simulink model "bh_4dof_LAGR_manipulator_CONTROL_PID"  (R2016b)
settings: Solver=ode15s  StartTime=0.0  StopTime=60  FixedStep=0.001  RelTol=1e-5  EnableMultiTasking=on
undefined symbols (not defined in the file or in its folder): b1_damp, b2_damp, b3_damp, b4_damp, g, Hz, L1x, L1y, L1z, L2x, L2y, L2z, L3x, L3y, L3z, mass1, mass2, mass3, mass4, Rturn, theta1_0, theta1_dot_0, theta2_0, theta2_dot_0, theta3_0, theta3_dot_0, theta4_0, theta4_dot_0, X, Y, Z
libraries: sm_lib x25, nesl_utility x17, simulink x9, simulink_extras x2
(part 2 of 3)

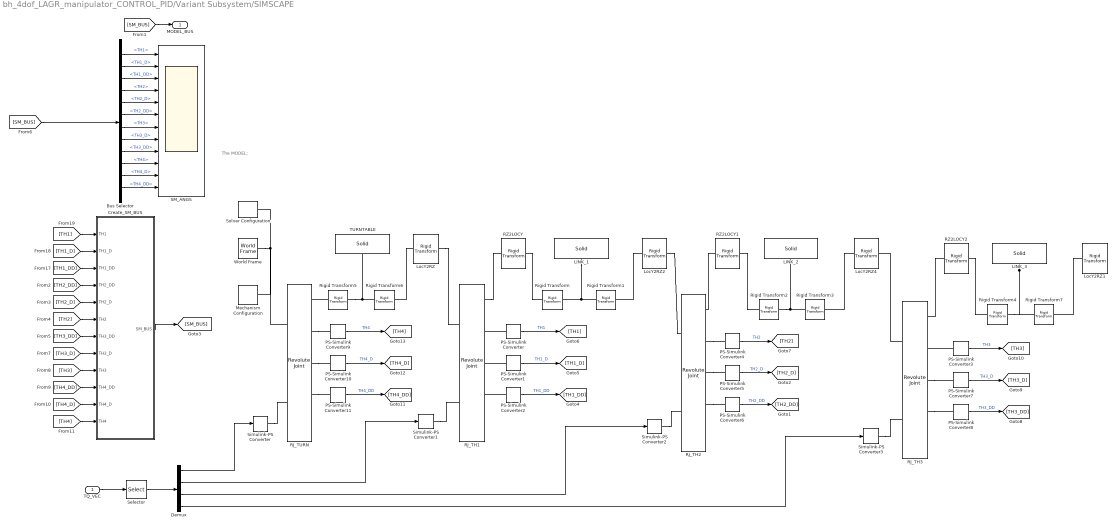
== system bh_4dof_LAGR_manipulator_CONTROL_PID/Variant Subsystem/SIMSCAPE ==
  note: The MODEL:
  TQ_VEC : Inport
  Bus Selector : BusSelector  OutputSignals=TH1,TH1_D,TH1_DD,TH2,TH2_D,TH2_DD,TH3,TH3_D,TH3_DD,TH4,TH4_D,TH4_DD
  Create_SM_BUS : Subsystem
  Demux : Demux
  LINK_1 : sm_lib/Body Elements/Solid  InertiaType=CalculateFromGeometry  Mass=1  MassUnits=kg  CenterOfMass=[0 0 0]  CenterOfMassUnits=m  MomentsOfInertia=[1 1 1]  MomentsOfInertiaUnits=kg*m^2  ProductsOfInertia=[0 0 0]  ProductsOfInertiaUnits=kg*m^2  DensityBased=on  Density=density  DensityUnits=kg/(m^3)  DoExposeReferenceFrame=on  SerializedFrames=<Frames/>  GraphicType=FromGeometry  MarkerShape=Sphere  MarkerSize=10  GraphicVisPropType=SimpleVisualProperties  GraphicDiffuseColor=[0.2 0.2 1.0]  GraphicSpecularColor=[0.5 0.5 0.5 1.0]  GraphicAmbientColor=[0.15 0.15 0.15 1.0]  GraphicEmissiveColor=[0.0 0.0 0.0 1.0]  GraphicShininess=75  GraphicOpacity=1.0  GeometryShape=Brick  RectangleSize=[1 1]  RectangleSizeUnits=m  BrickDimensions=[L1x, L1y, L1z ]  BrickDimensionUnits=m  CylinderRadius=1  CylinderRadiusUnits=m  CylinderLength=1  CylinderLengthUnits=m  SphereRadius=1  SphereRadiusUnits=m  EllipsoidRadii=[1 1 1]  EllipsoidRadiiUnits=m  ExtrusionCrossSection=[1 1; -1 1; -1 -1; 1 -1]  ExtrusionCrossSectionUnits=m  ExtrusionLength=1  ExtrusionLengthUnits=m  PolygonNumSides=3  PolygonOuterRadius=1  PolygonOuterRadiusUnits=m  ExtGeomFileType=STEP  ExtGeomFileUnits=m  RevolutionCrossSection=[1 1; 1 -1; 2 -1; 2 1]  RevolutionCrossSectionUnits=m  RevolutionExtent=Full  RevolutionAngle=180  RevolutionAngleUnits=deg
  LINK_2 : sm_lib/Body Elements/Solid  InertiaType=CalculateFromGeometry  Mass=1  MassUnits=kg  CenterOfMass=[0 0 0]  CenterOfMassUnits=m  MomentsOfInertia=[1 1 1]  MomentsOfInertiaUnits=kg*m^2  ProductsOfInertia=[0 0 0]  ProductsOfInertiaUnits=kg*m^2  DensityBased=on  Density=density  DensityUnits=kg/(m^3)  DoExposeReferenceFrame=on  SerializedFrames=<Frames/>  GraphicType=FromGeometry  MarkerShape=Sphere  MarkerSize=10  GraphicVisPropType=SimpleVisualProperties  GraphicDiffuseColor=[0.8 0.8 1.0]  GraphicSpecularColor=[0.5 0.5 0.5 1.0]  GraphicAmbientColor=[0.15 0.15 0.15 1.0]  GraphicEmissiveColor=[0.0 0.0 0.0 1.0]  GraphicShininess=75  GraphicOpacity=1.0  GeometryShape=Brick  RectangleSize=[1 1]  RectangleSizeUnits=m  BrickDimensions=[L2x, L2y, L2z ]  BrickDimensionUnits=m  CylinderRadius=1  CylinderRadiusUnits=m  CylinderLength=1  CylinderLengthUnits=m  SphereRadius=1  SphereRadiusUnits=m  EllipsoidRadii=[1 1 1]  EllipsoidRadiiUnits=m  ExtrusionCrossSection=[1 1; -1 1; -1 -1; 1 -1]  ExtrusionCrossSectionUnits=m  ExtrusionLength=1  ExtrusionLengthUnits=m  PolygonNumSides=3  PolygonOuterRadius=1  PolygonOuterRadiusUnits=m  ExtGeomFileType=STEP  ExtGeomFileUnits=m  RevolutionCrossSection=[1 1; 1 -1; 2 -1; 2 1]  RevolutionCrossSectionUnits=m  RevolutionExtent=Full  RevolutionAngle=180  RevolutionAngleUnits=deg
  LINK_3 : sm_lib/Body Elements/Solid  InertiaType=CalculateFromGeometry  Mass=1  MassUnits=kg  CenterOfMass=[0 0 0]  CenterOfMassUnits=m  MomentsOfInertia=[1 1 1]  MomentsOfInertiaUnits=kg*m^2  ProductsOfInertia=[0 0 0]  ProductsOfInertiaUnits=kg*m^2  DensityBased=on  Density=density  DensityUnits=kg/(m^3)  DoExposeReferenceFrame=on  SerializedFrames=<Frames/>  GraphicType=FromGeometry  MarkerShape=Sphere  MarkerSize=10  GraphicVisPropType=SimpleVisualProperties  GraphicDiffuseColor=[1.0 0.8 0.4]  GraphicSpecularColor=[0.5 0.5 0.5 1.0]  GraphicAmbientColor=[0.15 0.15 0.15 1.0]  GraphicEmissiveColor=[0.0 0.0 0.0 1.0]  GraphicShininess=75  GraphicOpacity=1.0  GeometryShape=Brick  RectangleSize=[1 1]  RectangleSizeUnits=m  BrickDimensions=[L3x, L3y, L3z ]  BrickDimensionUnits=m  CylinderRadius=1  CylinderRadiusUnits=m  CylinderLength=1  CylinderLengthUnits=m  SphereRadius=1  SphereRadiusUnits=m  EllipsoidRadii=[1 1 1]  EllipsoidRadiiUnits=m  ExtrusionCrossSection=[1 1; -1 1; -1 -1; 1 -1]  ExtrusionCrossSectionUnits=m  ExtrusionLength=1  ExtrusionLengthUnits=m  PolygonNumSides=3  PolygonOuterRadius=1  PolygonOuterRadiusUnits=m  ExtGeomFileType=STEP  ExtGeomFileUnits=m  RevolutionCrossSection=[1 1; 1 -1; 2 -1; 2 1]  RevolutionCrossSectionUnits=m  RevolutionExtent=Full  RevolutionAngle=180  RevolutionAngleUnits=deg
  LocY2RZ{,1..2,4} (4 alike) : sm_lib/Frames and Transforms/Rigid Transform  TranslationMethod=None  TranslationStandardOffset=Hz/2  TranslationLengthUnit=m  TranslationStandardAxis=+Z  TranslationCartesianOffset=[0 0 0]  TranslationROffset=0  TranslationROffsetUnits=m  TranslationZOffset=0  TranslationZOffsetUnits=m  TranslationThetaOffset=0  TranslationThetaOffsetUnits=deg  RotationMethod=AlignedAxes  RotationAngleUnits=deg  RotationStandardAxis=+Z  RotationAngle=0.0  RotationArbitraryAxis=[0 0 1]  FollAlignAxisA=+X  BaseAlignAxisA=+Y  FollAlignAxisB=+Y  BaseAlignAxisB=+Z  RotationSequenceAxes=FollowerAxes  RotationSequence=XYX  RotationSequenceAngles=[0 0 0]  RotationSequenceAnglesUnits=deg  RotationMatrix=[1 0 0; 0 1 0; 0 0 1]
  Mechanism Configuration : sm_lib/Utilities/Mechanism Configuration  UniformGravity=Constant  GravityVector=[0 0 -9.80665 ]  GravityUnits=m/s^2  LinearizationDelta=1e-4
  PS-Simulink Converter{,3..4,9} (4 alike) : nesl_utility/PS-Simulink Converter  PhysicalDomain=network_engine_domain  SubClassName=ps_output  LeftPortType=input  RightPortType=output  PseudoPeriodic=off  Frequencies=[]  Unit=rad  AffineConversion=off
  PS-Simulink Converter{1,5,7,10} (4 alike) : nesl_utility/PS-Simulink Converter  PhysicalDomain=network_engine_domain  SubClassName=ps_output  LeftPortType=input  RightPortType=output  PseudoPeriodic=off  Frequencies=[]  Unit=rad/s  AffineConversion=off
  PS-Simulink Converter{2,6,8,11} (4 alike) : nesl_utility/PS-Simulink Converter  PhysicalDomain=network_engine_domain  SubClassName=ps_output  LeftPortType=input  RightPortType=output  PseudoPeriodic=off  Frequencies=[]  Unit=rad/s^2  AffineConversion=off
  RJ_TH1 : sm_lib/Joints/Revolute Joint  SenseConstraintForce=on  SenseConstraintForceX=off  SenseConstraintForceY=off  SenseConstraintForceZ=off  SenseConstraintTorque=off  SenseConstraintTorqueX=off  SenseConstraintTorqueY=off  SenseConstraintTorqueZ=off  SenseTotalForce=off  SenseTotalForceX=off  SenseTotalForceY=off  SenseTotalForceZ=off  SenseTotalTorque=off  SenseTotalTorqueX=off  SenseTotalTorqueY=off  SenseTotalTorqueZ=off  CompositeWrenchDir=BaseOnFollower  CompositeWrenchFrame=BaseFrame  EquilibriumPosition=0  EquilibriumPositionUnits=deg  SpringStiffness=0  SpringStiffnessUnits=N*m/deg  DampingCoefficient=b1_damp  DampingCoefficientUnits=N*m/(rad/s)  TorqueActuationMode=InputTorque  MotionActuationMode=ComputedMotion  SensePosition=on  SenseVelocity=on  SenseAcceleration=on  SenseTorqueForce=off  PositionTargetSpecify=on  PositionTargetPriority=Low  PositionTargetValue=theta1_0  PositionTargetValueUnits=rad  VelocityTargetSpecify=on  VelocityTargetPriority=High  VelocityTargetValue=theta1_dot_0  VelocityTargetValueUnits=rad/s
      settings: AttributesFormatString=|
      | %<DampingCoefficient>
      | %<PositionTargetValue>
      | %<VelocityTargetValue>
  RJ_TH2 : sm_lib/Joints/Revolute Joint  SenseConstraintForce=on  SenseConstraintForceX=off  SenseConstraintForceY=off  SenseConstraintForceZ=off  SenseConstraintTorque=off  SenseConstraintTorqueX=off  SenseConstraintTorqueY=off  SenseConstraintTorqueZ=off  SenseTotalForce=off  SenseTotalForceX=off  SenseTotalForceY=off  SenseTotalForceZ=off  SenseTotalTorque=off  SenseTotalTorqueX=off  SenseTotalTorqueY=off  SenseTotalTorqueZ=off  CompositeWrenchDir=BaseOnFollower  CompositeWrenchFrame=BaseFrame  EquilibriumPosition=0  EquilibriumPositionUnits=deg  SpringStiffness=0  SpringStiffnessUnits=N*m/deg  DampingCoefficient=b2_damp  DampingCoefficientUnits=N*m/(rad/s)  TorqueActuationMode=InputTorque  MotionActuationMode=ComputedMotion  SensePosition=on  SenseVelocity=on  SenseAcceleration=on  SenseTorqueForce=off  PositionTargetSpecify=on  PositionTargetPriority=Low  PositionTargetValue=theta2_0  PositionTargetValueUnits=rad  VelocityTargetSpecify=on  VelocityTargetPriority=High  VelocityTargetValue=theta2_dot_0  VelocityTargetValueUnits=rad/s
      settings: AttributesFormatString=|
      | %<DampingCoefficient>
      | %<PositionTargetValue>
      | %<VelocityTargetValue>
  RJ_TH3 : sm_lib/Joints/Revolute Joint  SenseConstraintForce=on  SenseConstraintForceX=off  SenseConstraintForceY=off  SenseConstraintForceZ=off  SenseConstraintTorque=off  SenseConstraintTorqueX=off  SenseConstraintTorqueY=off  SenseConstraintTorqueZ=off  SenseTotalForce=off  SenseTotalForceX=off  SenseTotalForceY=off  SenseTotalForceZ=off  SenseTotalTorque=off  SenseTotalTorqueX=off  SenseTotalTorqueY=off  SenseTotalTorqueZ=off  CompositeWrenchDir=BaseOnFollower  CompositeWrenchFrame=BaseFrame  EquilibriumPosition=0  EquilibriumPositionUnits=deg  SpringStiffness=0  SpringStiffnessUnits=N*m/deg  DampingCoefficient=b3_damp  DampingCoefficientUnits=N*m/(rad/s)  TorqueActuationMode=InputTorque  MotionActuationMode=ComputedMotion  SensePosition=on  SenseVelocity=on  SenseAcceleration=on  SenseTorqueForce=off  PositionTargetSpecify=on  PositionTargetPriority=Low  PositionTargetValue=theta3_0  PositionTargetValueUnits=rad  VelocityTargetSpecify=on  VelocityTargetPriority=High  VelocityTargetValue=theta3_dot_0  VelocityTargetValueUnits=rad/s
      settings: AttributesFormatString=|
      | %<DampingCoefficient>
      | %<PositionTargetValue>
      | %<VelocityTargetValue>
  RJ_TURN : sm_lib/Joints/Revolute Joint  SenseConstraintForce=on  SenseConstraintForceX=off  SenseConstraintForceY=off  SenseConstraintForceZ=off  SenseConstraintTorque=off  SenseConstraintTorqueX=off  SenseConstraintTorqueY=off  SenseConstraintTorqueZ=off  SenseTotalForce=off  SenseTotalForceX=off  SenseTotalForceY=off  SenseTotalForceZ=off  SenseTotalTorque=off  SenseTotalTorqueX=off  SenseTotalTorqueY=off  SenseTotalTorqueZ=off  CompositeWrenchDir=BaseOnFollower  CompositeWrenchFrame=BaseFrame  EquilibriumPosition=0  EquilibriumPositionUnits=deg  SpringStiffness=0  SpringStiffnessUnits=N*m/deg  DampingCoefficient=b4_damp  DampingCoefficientUnits=N*m/(rad/s)  TorqueActuationMode=InputTorque  MotionActuationMode=ComputedMotion  SensePosition=on  SenseVelocity=on  SenseAcceleration=on  SenseTorqueForce=off  PositionTargetSpecify=on  PositionTargetPriority=Low  PositionTargetValue=theta4_0  PositionTargetValueUnits=rad  VelocityTargetSpecify=on  VelocityTargetPriority=High  VelocityTargetValue=theta4_dot_0  VelocityTargetValueUnits=rad/s
      settings: AttributesFormatString=|
      | %<DampingCoefficient>
      | %<PositionTargetValue>
      | %<VelocityTargetValue>
  RZ2LOCY : sm_lib/Frames and Transforms/Rigid Transform  TranslationMethod=None  TranslationStandardOffset=Hz/2  TranslationLengthUnit=m  TranslationStandardAxis=+Z  TranslationCartesianOffset=[0 0 0]  TranslationROffset=0  TranslationROffsetUnits=m  TranslationZOffset=0  TranslationZOffsetUnits=m  TranslationThetaOffset=0  TranslationThetaOffsetUnits=deg  RotationMethod=AlignedAxes  RotationAngleUnits=deg  RotationStandardAxis=+Z  RotationAngle=0.0  RotationArbitraryAxis=[0 0 1]  FollAlignAxisA=+Y  BaseAlignAxisA=+X  FollAlignAxisB=+X  BaseAlignAxisB=+Z  RotationSequenceAxes=FollowerAxes  RotationSequence=XYX  RotationSequenceAngles=[0 0 0]  RotationSequenceAnglesUnits=deg  RotationMatrix=[1 0 0; 0 1 0; 0 0 1]
  RZ2LOCY1 : sm_lib/Frames and Transforms/Rigid Transform  TranslationMethod=None  TranslationStandardOffset=Hz/2  TranslationLengthUnit=m  TranslationStandardAxis=+Z  TranslationCartesianOffset=[0 0 0]  TranslationROffset=0  TranslationROffsetUnits=m  TranslationZOffset=0  TranslationZOffsetUnits=m  TranslationThetaOffset=0  TranslationThetaOffsetUnits=deg  RotationMethod=AlignedAxes  RotationAngleUnits=deg  RotationStandardAxis=+Z  RotationAngle=0.0  RotationArbitraryAxis=[0 0 1]  FollAlignAxisA=+Y  BaseAlignAxisA=+X  FollAlignAxisB=+X  BaseAlignAxisB=+Z  RotationSequenceAxes=FollowerAxes  RotationSequence=XYX  RotationSequenceAngles=[0 0 0]  RotationSequenceAnglesUnits=deg  RotationMatrix=[1 0 0; 0 1 0; 0 0 1]
  RZ2LOCY2 : sm_lib/Frames and Transforms/Rigid Transform  TranslationMethod=None  TranslationStandardOffset=Hz/2  TranslationLengthUnit=m  TranslationStandardAxis=+Z  TranslationCartesianOffset=[0 0 0]  TranslationROffset=0  TranslationROffsetUnits=m  TranslationZOffset=0  TranslationZOffsetUnits=m  TranslationThetaOffset=0  TranslationThetaOffsetUnits=deg  RotationMethod=AlignedAxes  RotationAngleUnits=deg  RotationStandardAxis=+Z  RotationAngle=0.0  RotationArbitraryAxis=[0 0 1]  FollAlignAxisA=+Y  BaseAlignAxisA=+X  FollAlignAxisB=+X  BaseAlignAxisB=+Z  RotationSequenceAxes=FollowerAxes  RotationSequence=XYX  RotationSequenceAngles=[0 0 0]  RotationSequenceAnglesUnits=deg  RotationMatrix=[1 0 0; 0 1 0; 0 0 1]
  Rigid Transform : sm_lib/Frames and Transforms/Rigid Transform  TranslationMethod=StandardAxis  TranslationStandardOffset=L1y/2  TranslationLengthUnit=m  TranslationStandardAxis=+Y  TranslationCartesianOffset=[0 0 0]  TranslationROffset=0  TranslationROffsetUnits=m  TranslationZOffset=0  TranslationZOffsetUnits=m  TranslationThetaOffset=0  TranslationThetaOffsetUnits=deg  RotationMethod=None  RotationAngleUnits=deg  RotationStandardAxis=+Z  RotationAngle=0.0  RotationArbitraryAxis=[0 0 1]  FollAlignAxisA=+X  BaseAlignAxisA=+Y  FollAlignAxisB=+Y  BaseAlignAxisB=+Z  RotationSequenceAxes=FollowerAxes  RotationSequence=XYX  RotationSequenceAngles=[0 0 0]  RotationSequenceAnglesUnits=deg  RotationMatrix=[1 0 0; 0 1 0; 0 0 1]
  Rigid Transform1 : sm_lib/Frames and Transforms/Rigid Transform  TranslationMethod=StandardAxis  TranslationStandardOffset=L1y/2  TranslationLengthUnit=m  TranslationStandardAxis=+Y  TranslationCartesianOffset=[0 0 0]  TranslationROffset=0  TranslationROffsetUnits=m  TranslationZOffset=0  TranslationZOffsetUnits=m  TranslationThetaOffset=0  TranslationThetaOffsetUnits=deg  RotationMethod=None  RotationAngleUnits=deg  RotationStandardAxis=+Z  RotationAngle=0.0  RotationArbitraryAxis=[0 0 1]  FollAlignAxisA=+X  BaseAlignAxisA=+Y  FollAlignAxisB=+Y  BaseAlignAxisB=+Z  RotationSequenceAxes=FollowerAxes  RotationSequence=XYX  RotationSequenceAngles=[0 0 0]  RotationSequenceAnglesUnits=deg  RotationMatrix=[1 0 0; 0 1 0; 0 0 1]
  Rigid Transform2 : sm_lib/Frames and Transforms/Rigid Transform  TranslationMethod=StandardAxis  TranslationStandardOffset=L2y/2  TranslationLengthUnit=m  TranslationStandardAxis=+Y  TranslationCartesianOffset=[0 0 0]  TranslationROffset=0  TranslationROffsetUnits=m  TranslationZOffset=0  TranslationZOffsetUnits=m  TranslationThetaOffset=0  TranslationThetaOffsetUnits=deg  RotationMethod=None  RotationAngleUnits=deg  RotationStandardAxis=+Z  RotationAngle=0.0  RotationArbitraryAxis=[0 0 1]  FollAlignAxisA=+X  BaseAlignAxisA=+Y  FollAlignAxisB=+Y  BaseAlignAxisB=+Z  RotationSequenceAxes=FollowerAxes  RotationSequence=XYX  RotationSequenceAngles=[0 0 0]  RotationSequenceAnglesUnits=deg  RotationMatrix=[1 0 0; 0 1 0; 0 0 1]
  Rigid Transform3 : sm_lib/Frames and Transforms/Rigid Transform  TranslationMethod=StandardAxis  TranslationStandardOffset=L2y/2  TranslationLengthUnit=m  TranslationStandardAxis=+Y  TranslationCartesianOffset=[0 0 0]  TranslationROffset=0  TranslationROffsetUnits=m  TranslationZOffset=0  TranslationZOffsetUnits=m  TranslationThetaOffset=0  TranslationThetaOffsetUnits=deg  RotationMethod=None  RotationAngleUnits=deg  RotationStandardAxis=+Z  RotationAngle=0.0  RotationArbitraryAxis=[0 0 1]  FollAlignAxisA=+X  BaseAlignAxisA=+Y  FollAlignAxisB=+Y  BaseAlignAxisB=+Z  RotationSequenceAxes=FollowerAxes  RotationSequence=XYX  RotationSequenceAngles=[0 0 0]  RotationSequenceAnglesUnits=deg  RotationMatrix=[1 0 0; 0 1 0; 0 0 1]
  Rigid Transform4 : sm_lib/Frames and Transforms/Rigid Transform  TranslationMethod=StandardAxis  TranslationStandardOffset=L3y/2  TranslationLengthUnit=m  TranslationStandardAxis=+Y  TranslationCartesianOffset=[0 0 0]  TranslationROffset=0  TranslationROffsetUnits=m  TranslationZOffset=0  TranslationZOffsetUnits=m  TranslationThetaOffset=0  TranslationThetaOffsetUnits=deg  RotationMethod=None  RotationAngleUnits=deg  RotationStandardAxis=+Z  RotationAngle=0.0  RotationArbitraryAxis=[0 0 1]  FollAlignAxisA=+X  BaseAlignAxisA=+Y  FollAlignAxisB=+Y  BaseAlignAxisB=+Z  RotationSequenceAxes=FollowerAxes  RotationSequence=XYX  RotationSequenceAngles=[0 0 0]  RotationSequenceAnglesUnits=deg  RotationMatrix=[1 0 0; 0 1 0; 0 0 1]
  Rigid Transform5 : sm_lib/Frames and Transforms/Rigid Transform  TranslationMethod=StandardAxis  TranslationStandardOffset=Hz/2  TranslationLengthUnit=m  TranslationStandardAxis=-Z  TranslationCartesianOffset=[0 0 0]  TranslationROffset=0  TranslationROffsetUnits=m  TranslationZOffset=0  TranslationZOffsetUnits=m  TranslationThetaOffset=0  TranslationThetaOffsetUnits=deg  RotationMethod=None  RotationAngleUnits=deg  RotationStandardAxis=+Z  RotationAngle=0.0  RotationArbitraryAxis=[0 0 1]  FollAlignAxisA=+X  BaseAlignAxisA=+Y  FollAlignAxisB=+Y  BaseAlignAxisB=+Z  RotationSequenceAxes=FollowerAxes  RotationSequence=XYX  RotationSequenceAngles=[0 0 0]  RotationSequenceAnglesUnits=deg  RotationMatrix=[1 0 0; 0 1 0; 0 0 1]
  Rigid Transform6 : sm_lib/Frames and Transforms/Rigid Transform  TranslationMethod=StandardAxis  TranslationStandardOffset=Hz/2  TranslationLengthUnit=m  TranslationStandardAxis=+Z  TranslationCartesianOffset=[0 0 0]  TranslationROffset=0  TranslationROffsetUnits=m  TranslationZOffset=0  TranslationZOffsetUnits=m  TranslationThetaOffset=0  TranslationThetaOffsetUnits=deg  RotationMethod=None  RotationAngleUnits=deg  RotationStandardAxis=+Z  RotationAngle=0.0  RotationArbitraryAxis=[0 0 1]  FollAlignAxisA=+X  BaseAlignAxisA=+Y  FollAlignAxisB=+Y  BaseAlignAxisB=+Z  RotationSequenceAxes=FollowerAxes  RotationSequence=XYX  RotationSequenceAngles=[0 0 0]  RotationSequenceAnglesUnits=deg  RotationMatrix=[1 0 0; 0 1 0; 0 0 1]
  Rigid Transform7 : sm_lib/Frames and Transforms/Rigid Transform  TranslationMethod=StandardAxis  TranslationStandardOffset=L3y/2  TranslationLengthUnit=m  TranslationStandardAxis=+Y  TranslationCartesianOffset=[0 0 0]  TranslationROffset=0  TranslationROffsetUnits=m  TranslationZOffset=0  TranslationZOffsetUnits=m  TranslationThetaOffset=0  TranslationThetaOffsetUnits=deg  RotationMethod=None  RotationAngleUnits=deg  RotationStandardAxis=+Z  RotationAngle=0.0  RotationArbitraryAxis=[0 0 1]  FollAlignAxisA=+X  BaseAlignAxisA=+Y  FollAlignAxisB=+Y  BaseAlignAxisB=+Z  RotationSequenceAxes=FollowerAxes  RotationSequence=XYX  RotationSequenceAngles=[0 0 0]  RotationSequenceAnglesUnits=deg  RotationMatrix=[1 0 0; 0 1 0; 0 0 1]
  SM_ANGS : Scope  NumInputPorts=12
  Selector : Selector  InputPortWidth=4  IndexOptions=Index vector (dialog)  Indices=[4 1 2 3]  OutputSizes=1
  Simulink-PS Converter{,1..3} (4 alike) : nesl_utility/Simulink-PS Converter  PhysicalDomain=network_engine_domain  SubClassName=ps_input  LeftPortType=input  RightPortType=output  PseudoPeriodic=off  Frequencies=[]  NoiseDistribution=none  NoiseParameters=[]  Unit=N*m  AffineConversion=off  InputFiltering=off  SimscapeFilterOrder=1  InputFilterTimeConstant=0.001  UdotUserProvided=1
  Solver Configuration : nesl_utility/Solver Configuration  PhysicalDomain=network_engine_domain  SubClassName=solver  LeftPortType=input  RightPortType=generic  Accelerate=off  Tones=[]  Harmonics=[]  SimulateNoise=off  Profile=off  UseLocalSampling=off  EnableSwitchedLinearOptims=on  FrequencyDomain=off  UseCCode=off  RelTol=0.001  AbsTol=1e-06  MinStep=1e-09  ToWorkspace=off  RevertToSquareIcSolve=off  NumHomotopyIterations=100  PhasorMode=off  PhasorModeNumHarmonics=1  OverrideAbsTol=off  DoDC=off  ResidualTolerance=1e-09  UseLocalSolver=off  LocalSolverChoice=NE_TRAPEZOIDAL_ADVANCER  LocalSolverSampleTime=0.01  DoFixedCost=off  MaxNonlinIter=3  MaxModeIter=2  LinearAlgebra=Sparse  DelaysMemoryBudget=1024  AutomaticFiltering=off  FilteringTimeConstant=0.001
  TURNTABLE : sm_lib/Body Elements/Solid  InertiaType=CalculateFromGeometry  Mass=1  MassUnits=kg  CenterOfMass=[0 0 0]  CenterOfMassUnits=m  MomentsOfInertia=[1 1 1]  MomentsOfInertiaUnits=kg*m^2  ProductsOfInertia=[0 0 0]  ProductsOfInertiaUnits=kg*m^2  DensityBased=on  Density=1000  DensityUnits=kg/(m^3)  DoExposeReferenceFrame=on  SerializedFrames=<Frames/>  GraphicType=FromGeometry  MarkerShape=Sphere  MarkerSize=10  GraphicVisPropType=SimpleVisualProperties  GraphicDiffuseColor=[1.0 1.0 0.2]  GraphicSpecularColor=[0.5 0.5 0.5 1.0]  GraphicAmbientColor=[0.15 0.15 0.15 1.0]  GraphicEmissiveColor=[0.0 0.0 0.0 1.0]  GraphicShininess=75  GraphicOpacity=1.0  GeometryShape=Cylinder  RectangleSize=[1 1]  RectangleSizeUnits=m  BrickDimensions=[1 1 1]  BrickDimensionUnits=m  CylinderRadius=Rturn  CylinderRadiusUnits=m  CylinderLength=Hz  CylinderLengthUnits=m  SphereRadius=1  SphereRadiusUnits=m  EllipsoidRadii=[1 1 1]  EllipsoidRadiiUnits=m  ExtrusionCrossSection=[1 1; -1 1; -1 -1; 1 -1]  ExtrusionCrossSectionUnits=m  ExtrusionLength=1  ExtrusionLengthUnits=m  PolygonNumSides=3  PolygonOuterRadius=1  PolygonOuterRadiusUnits=m  ExtGeomFileType=STEP  ExtGeomFileUnits=m  RevolutionCrossSection=[1 1; 1 -1; 2 -1; 2 1]  RevolutionCrossSectionUnits=m  RevolutionExtent=Full  RevolutionAngle=180  RevolutionAngleUnits=deg
  World Frame : sm_lib/Frames and Transforms/World Frame
  MODEL_BUS : Outport
  wires:
  [SM_BUS] -> MODEL_BUS/1
  [TH2_D] -> Create_SM_BUS/5(TH2_D)
  [TH1_D] -> Create_SM_BUS/2(TH1_D)
  [TH2_DD] -> Create_SM_BUS/4(TH2_DD)
  [TH2] -> Create_SM_BUS/6(TH2)
  [TH1_DD] -> Create_SM_BUS/3(TH1_DD)
  [TH1] -> Create_SM_BUS/1(TH1)
  Create_SM_BUS/1(SM_BUS) -> [SM_BUS]
  Bus Selector/2 -> SM_ANGS/2  "<TH1_D>"
  Bus Selector/3 -> SM_ANGS/3  "<TH1_DD>"
  Bus Selector/1 -> SM_ANGS/1  "<TH1>"
  Bus Selector/4 -> SM_ANGS/4  "<TH2>"
  Bus Selector/5 -> SM_ANGS/5  "<TH2_D>"
  Bus Selector/6 -> SM_ANGS/6  "<TH2_DD>"
  Bus Selector/7 -> SM_ANGS/7  "<TH3>"
  Bus Selector/8 -> SM_ANGS/8  "<TH3_D>"
  Bus Selector/9 -> SM_ANGS/9  "<TH3_DD>"
  [TH3_DD] -> Create_SM_BUS/7(TH3_DD)
  [TH3_D] -> Create_SM_BUS/8(TH3_D)
  [TH3] -> Create_SM_BUS/9(TH3)
  PS-Simulink Converter/1 -> [TH1]  "TH1"
  PS-Simulink Converter2/1 -> [TH1_DD]  "TH1_DD"
  PS-Simulink Converter1/1 -> [TH1_D]  "TH1_D"
  PS-Simulink Converter4/1 -> [TH2]  "TH2"
  PS-Simulink Converter6/1 -> [TH2_DD]  "TH2_DD"
  PS-Simulink Converter5/1 -> [TH2_D]  "TH2_D"
  PS-Simulink Converter3/1 -> [TH3]  "TH3"
  PS-Simulink Converter8/1 -> [TH3_DD]  "TH3_DD"
  PS-Simulink Converter7/1 -> [TH3_D]  "TH3_D"
  PS-Simulink Converter9/1 -> [TH4]  "TH4"
  PS-Simulink Converter11/1 -> [TH4_DD]  "TH4_DD"
  PS-Simulink Converter10/1 -> [TH4_D]  "TH4_D"
  [TH4_DD] -> Create_SM_BUS/10(TH4_DD)
  [TH4_D] -> Create_SM_BUS/11(TH4_D)
  [TH4] -> Create_SM_BUS/12(TH4)
  Bus Selector/12 -> SM_ANGS/12  "<TH4_DD>"
  Bus Selector/11 -> SM_ANGS/11  "<TH4_D>"
  Bus Selector/10 -> SM_ANGS/10  "<TH4>"
  [SM_BUS] -> Bus Selector/1
  Demux/1 -> Simulink-PS Converter/1
  Demux/2 -> Simulink-PS Converter1/1
  Demux/3 -> Simulink-PS Converter2/1
  Demux/4 -> Simulink-PS Converter3/1
  TQ_VEC/1 -> Selector/1
  Selector/1 -> Demux/1
  connections:
  World Frame/RConn1 -- RJ_TURN/LConn1 -- Mechanism Configuration/RConn1 -- Solver Configuration/RConn1
  PS-Simulink Converter1/LConn1 -- RJ_TH1/RConn3
  PS-Simulink Converter2/LConn1 -- RJ_TH1/RConn4
  PS-Simulink Converter/LConn1 -- RJ_TH1/RConn2
  Rigid Transform5/LConn1 -- RJ_TURN/RConn1
  Rigid Transform5/RConn1 -- Rigid Transform6/LConn1 -- TURNTABLE/RConn1
  LocY2RZ/LConn1 -- Rigid Transform6/RConn1
  LocY2RZ/RConn1 -- RJ_TH1/LConn1
  Rigid Transform1/LConn1 -- LINK_1/RConn1 -- Rigid Transform/RConn1
  LocY2RZ2/LConn1 -- Rigid Transform1/RConn1
  LocY2RZ2/RConn1 -- RJ_TH2/LConn1
  RZ2LOCY1/LConn1 -- RJ_TH2/RConn1
  Rigid Transform2/RConn1 -- Rigid Transform3/LConn1 -- LINK_2/RConn1
  LocY2RZ4/LConn1 -- Rigid Transform3/RConn1
  RJ_TH1/RConn1 -- RZ2LOCY/LConn1
  RZ2LOCY/RConn1 -- Rigid Transform/LConn1
  RZ2LOCY1/RConn1 -- Rigid Transform2/LConn1
  RJ_TH3/LConn1 -- LocY2RZ4/RConn1
  LINK_3/RConn1 -- Rigid Transform7/LConn1 -- Rigid Transform4/RConn1
  LocY2RZ1/LConn1 -- Rigid Transform7/RConn1
  RZ2LOCY2/RConn1 -- Rigid Transform4/LConn1
  RZ2LOCY2/LConn1 -- RJ_TH3/RConn1
  RJ_TH2/RConn3 -- PS-Simulink Converter5/LConn1
  RJ_TH2/RConn2 -- PS-Simulink Converter4/LConn1
  RJ_TH2/RConn4 -- PS-Simulink Converter6/LConn1
  PS-Simulink Converter3/LConn1 -- RJ_TH3/RConn2
  RJ_TH3/RConn3 -- PS-Simulink Converter7/LConn1
  RJ_TH3/RConn4 -- PS-Simulink Converter8/LConn1
  RJ_TURN/RConn4 -- PS-Simulink Converter11/LConn1
  RJ_TURN/RConn3 -- PS-Simulink Converter10/LConn1
  RJ_TURN/RConn2 -- PS-Simulink Converter9/LConn1
  Simulink-PS Converter/RConn1 -- RJ_TURN/LConn2
  Simulink-PS Converter2/RConn1 -- RJ_TH2/LConn2
  Simulink-PS Converter3/RConn1 -- RJ_TH3/LConn2
  Simulink-PS Converter1/RConn1 -- RJ_TH1/LConn2

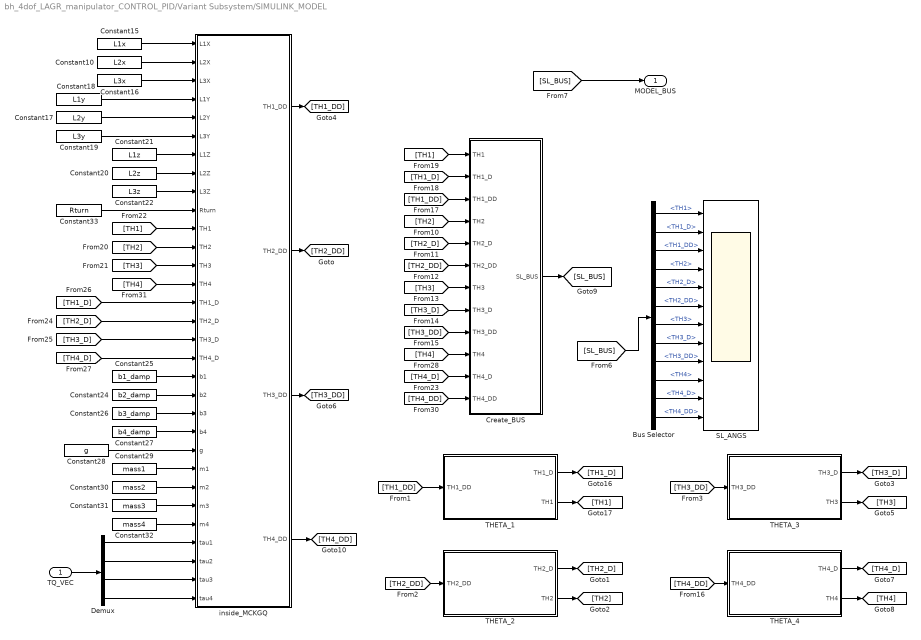
== system bh_4dof_LAGR_manipulator_CONTROL_PID/Variant Subsystem/SIMULINK_MODEL ==
  TQ_VEC : Inport
  Bus Selector : BusSelector  OutputSignals=TH1,TH1_D,TH1_DD,TH2,TH2_D,TH2_DD,TH3,TH3_D,TH3_DD,TH4,TH4_D,TH4_DD
  Constant10 : Constant  Value=L2x
  Constant15 : Constant  Value=L1x
  Constant16 : Constant  Value=L3x
  Constant17 : Constant  Value=L2y
  Constant18 : Constant  Value=L1y
  Constant19 : Constant  Value=L3y
  Constant20 : Constant  Value=L2z
  Constant21 : Constant  Value=L1z
  Constant22 : Constant  Value=L3z
  Constant24 : Constant  Value=b2_damp
  Constant25 : Constant  Value=b1_damp
  Constant26 : Constant  Value=b3_damp
  Constant27 : Constant  Value=b4_damp
  Constant28 : Constant  Value=g
  Constant29 : Constant  Value=mass1
  Constant30 : Constant  Value=mass2
  Constant31 : Constant  Value=mass3
  Constant32 : Constant  Value=mass4
  Constant33 : Constant  Value=Rturn
  Create_BUS : Subsystem
  Demux : Demux
  SL_ANGS : Scope  NumInputPorts=12
  THETA_1 : Subsystem
  THETA_2 : Subsystem
  THETA_3 : Subsystem
  THETA_4 : Subsystem
  inside_MCKGQ : Subsystem
  MODEL_BUS : Outport
  wires:
  [SL_BUS] -> Bus Selector/1
  Create_BUS/1(SL_BUS) -> [SL_BUS]
  Bus Selector/2 -> SL_ANGS/2  "<TH1_D>"
  Bus Selector/3 -> SL_ANGS/3  "<TH1_DD>"
  Bus Selector/1 -> SL_ANGS/1  "<TH1>"
  Bus Selector/4 -> SL_ANGS/4  "<TH2>"
  Bus Selector/5 -> SL_ANGS/5  "<TH2_D>"
  Bus Selector/6 -> SL_ANGS/6  "<TH2_DD>"
  Bus Selector/7 -> SL_ANGS/7  "<TH3>"
  Bus Selector/8 -> SL_ANGS/8  "<TH3_D>"
  Bus Selector/9 -> SL_ANGS/9  "<TH3_DD>"
  [TH2_DD] -> THETA_2/1(TH2_DD)
  THETA_2/2(TH2) -> [TH2]
  THETA_2/1(TH2_D) -> [TH2_D]
  [TH1_DD] -> THETA_1/1(TH1_DD)
  THETA_1/1(TH1_D) -> [TH1_D]
  THETA_1/2(TH1) -> [TH1]
  inside_MCKGQ/2(TH2_DD) -> [TH2_DD]
  [TH3_DD] -> THETA_3/1(TH3_DD)
  THETA_3/2(TH3) -> [TH3]
  THETA_3/1(TH3_D) -> [TH3_D]
  inside_MCKGQ/1(TH1_DD) -> [TH1_DD]
  inside_MCKGQ/3(TH3_DD) -> [TH3_DD]
  [TH3_DD] -> Create_BUS/9(TH3_DD)
  [TH1] -> Create_BUS/1(TH1)
  [TH1_D] -> Create_BUS/2(TH1_D)
  [TH1_DD] -> Create_BUS/3(TH1_DD)
  [TH2] -> Create_BUS/4(TH2)
  [TH2_D] -> Create_BUS/5(TH2_D)
  [TH2_DD] -> Create_BUS/6(TH2_DD)
  [TH3] -> Create_BUS/7(TH3)
  [TH3_D] -> Create_BUS/8(TH3_D)
  [TH4_DD] -> THETA_4/1(TH4_DD)
  THETA_4/2(TH4) -> [TH4]
  THETA_4/1(TH4_D) -> [TH4_D]
  [TH2] -> inside_MCKGQ/12(TH2)
  [TH3] -> inside_MCKGQ/13(TH3)
  [TH1] -> inside_MCKGQ/11(TH1)
  Constant10/1 -> inside_MCKGQ/2(L2X)
  Constant16/1 -> inside_MCKGQ/3(L3X)
  Constant15/1 -> inside_MCKGQ/1(L1X)
  Constant19/1 -> inside_MCKGQ/6(L3Y)
  Constant17/1 -> inside_MCKGQ/5(L2Y)
  Constant18/1 -> inside_MCKGQ/4(L1Y)
  Constant22/1 -> inside_MCKGQ/9(L3Z)
  Constant20/1 -> inside_MCKGQ/8(L2Z)
  Constant21/1 -> inside_MCKGQ/7(L1Z)
  [TH1_D] -> inside_MCKGQ/15(TH1_D)
  [TH2_D] -> inside_MCKGQ/16(TH2_D)
  [TH3_D] -> inside_MCKGQ/17(TH3_D)
  [TH4_D] -> inside_MCKGQ/18(TH4_D)
  Constant25/1 -> inside_MCKGQ/19(b1)
  Constant24/1 -> inside_MCKGQ/20(b2)
  Constant26/1 -> inside_MCKGQ/21(b3)
  Constant27/1 -> inside_MCKGQ/22(b4)
  Constant28/1 -> inside_MCKGQ/23(g)
  Constant29/1 -> inside_MCKGQ/24(m1)
  Constant30/1 -> inside_MCKGQ/25(m2)
  Constant31/1 -> inside_MCKGQ/26(m3)
  Constant32/1 -> inside_MCKGQ/27(m4)
  Constant33/1 -> inside_MCKGQ/10(Rturn)
  [TH4_D] -> Create_BUS/11(TH4_D)
  [TH4_DD] -> Create_BUS/12(TH4_DD)
  [TH4] -> Create_BUS/10(TH4)
  [TH4] -> inside_MCKGQ/14(TH4)
  inside_MCKGQ/4(TH4_DD) -> [TH4_DD]
  Bus Selector/10 -> SL_ANGS/10  "<TH4>"
  Bus Selector/11 -> SL_ANGS/11  "<TH4_D>"
  Bus Selector/12 -> SL_ANGS/12  "<TH4_DD>"
  [SL_BUS] -> MODEL_BUS/1
  Demux/1 -> inside_MCKGQ/28(tau1)
  Demux/2 -> inside_MCKGQ/29(tau2)
  Demux/3 -> inside_MCKGQ/30(tau3)
  Demux/4 -> inside_MCKGQ/31(tau4)
  TQ_VEC/1 -> Demux/1

== system bh_4dof_LAGR_manipulator_CONTROL_PID/Create_PLANT_BUS/Subsystem1/Subsystem1 ==
  mg_signed : Inport
  Constant : Constant  Value=0
  Mux : Mux  Inputs=3
  Reshape : Reshape  OutputDimensionality=Column vector (2-D)
  COL : Outport
  wires:
  mg_signed/1 -> Mux/3
  Constant/1 -> Mux/2, Mux/1
  Mux/1 -> Reshape/1
  Reshape/1 -> COL/1

== system bh_4dof_LAGR_manipulator_CONTROL_PID/Create_PLANT_BUS/Subsystem1/Subsystem2 ==
  mg_signed : Inport
  Constant : Constant  Value=0
  Mux : Mux  Inputs=3
  Reshape : Reshape  OutputDimensionality=Column vector (2-D)
  COL : Outport
  wires:
  mg_signed/1 -> Mux/3
  Constant/1 -> Mux/2, Mux/1
  Mux/1 -> Reshape/1
  Reshape/1 -> COL/1

== system bh_4dof_LAGR_manipulator_CONTROL_PID/Create_PLANT_BUS/Subsystem1/Subsystem3 ==
  mg_signed : Inport
  Constant : Constant  Value=0
  Mux : Mux  Inputs=3
  Reshape : Reshape  OutputDimensionality=Column vector (2-D)
  COL : Outport
  wires:
  mg_signed/1 -> Mux/3
  Constant/1 -> Mux/2, Mux/1
  Mux/1 -> Reshape/1
  Reshape/1 -> COL/1

== system bh_4dof_LAGR_manipulator_CONTROL_PID/Create_PLANT_BUS/Subsystem1/Subsystem4 ==
  mg_signed : Inport
  Constant : Constant  Value=0
  Mux : Mux  Inputs=3
  Reshape : Reshape  OutputDimensionality=Column vector (2-D)
  COL : Outport
  wires:
  mg_signed/1 -> Mux/3
  Constant/1 -> Mux/2, Mux/1
  Mux/1 -> Reshape/1
  Reshape/1 -> COL/1

== system bh_4dof_LAGR_manipulator_CONTROL_PID/Create_PLANT_BUS/Subsystem1/Subsystem5 ==
  mg_signed : Inport
  Constant : Constant  Value=0
  Mux : Mux  Inputs=3
  Reshape : Reshape  OutputDimensionality=Column vector (2-D)
  COL : Outport
  wires:
  mg_signed/1 -> Mux/3
  Constant/1 -> Mux/2, Mux/1
  Mux/1 -> Reshape/1
  Reshape/1 -> COL/1

== system bh_4dof_LAGR_manipulator_CONTROL_PID/Create_PLANT_BUS/Subsystem1/Subsystem6 ==
  mg_signed : Inport
  Constant : Constant  Value=0
  Mux : Mux  Inputs=3
  Reshape : Reshape  OutputDimensionality=Column vector (2-D)
  COL : Outport
  wires:
  mg_signed/1 -> Mux/3
  Constant/1 -> Mux/2, Mux/1
  Mux/1 -> Reshape/1
  Reshape/1 -> COL/1

== system bh_4dof_LAGR_manipulator_CONTROL_PID/Variant Subsystem/SIMSCAPE/Create_SM_BUS ==
  TH1 : Inport
  TH1_D : Inport  Port=2
  TH1_DD : Inport  Port=3
  TH2_DD : Inport  Port=4
  TH2_D : Inport  Port=5
  TH2 : Inport  Port=6
  TH3_DD : Inport  Port=7
  TH3_D : Inport  Port=8
  TH3 : Inport  Port=9
  TH4_DD : Inport  Port=10
  TH4_D : Inport  Port=11
  TH4 : Inport  Port=12
  Bus Creator : BusCreator  Inputs=12
  SM_BUS : Outport
  wires:
  TH2_DD/1 -> Bus Creator/4  "TH2_DD"
  TH1_DD/1 -> Bus Creator/3  "TH1_DD"
  TH1_D/1 -> Bus Creator/2  "TH1_D"
  TH2_D/1 -> Bus Creator/5  "TH2_D"
  TH1/1 -> Bus Creator/1  "TH1"
  TH2/1 -> Bus Creator/6  "TH2"
  Bus Creator/1 -> SM_BUS/1
  TH3/1 -> Bus Creator/9  "TH3"
  TH3_D/1 -> Bus Creator/8  "TH3_D"
  TH3_DD/1 -> Bus Creator/7  "TH3_DD"
  TH4/1 -> Bus Creator/12  "TH4"
  TH4_D/1 -> Bus Creator/11  "TH4_D"
  TH4_DD/1 -> Bus Creator/10  "TH4_DD"

== system bh_4dof_LAGR_manipulator_CONTROL_PID/Variant Subsystem/SIMULINK_MODEL/Create_BUS ==
  TH1 : Inport
  TH1_D : Inport  Port=2
  TH1_DD : Inport  Port=3
  TH2 : Inport  Port=4
  TH2_D : Inport  Port=5
  TH2_DD : Inport  Port=6
  TH3 : Inport  Port=7
  TH3_D : Inport  Port=8
  TH3_DD : Inport  Port=9
  TH4 : Inport  Port=10
  TH4_D : Inport  Port=11
  TH4_DD : Inport  Port=12
  Bus Creator : BusCreator  Inputs=12
  SL_BUS : Outport
  wires:
  TH1_DD/1 -> Bus Creator/3  "TH1_DD"
  TH1_D/1 -> Bus Creator/2  "TH1_D"
  TH1/1 -> Bus Creator/1  "TH1"
  Bus Creator/1 -> SL_BUS/1
  TH2/1 -> Bus Creator/4  "TH2"
  TH2_D/1 -> Bus Creator/5  "TH2_D"
  TH2_DD/1 -> Bus Creator/6  "TH2_DD"
  TH3/1 -> Bus Creator/7  "TH3"
  TH3_DD/1 -> Bus Creator/9  "TH3_DD"
  TH3_D/1 -> Bus Creator/8  "TH3_D"
  TH4_DD/1 -> Bus Creator/12  "TH4_DD"
  TH4_D/1 -> Bus Creator/11  "TH4_D"
  TH4/1 -> Bus Creator/10  "TH4"

== system bh_4dof_LAGR_manipulator_CONTROL_PID/Variant Subsystem/SIMULINK_MODEL/THETA_1 ==
  TH1_DD : Inport
  Constant15 : Constant  Value=theta1_0
  Constant16 : Constant  Value=theta1_dot_0
  Integrator2 : Integrator  InitialConditionSource=external
  Integrator3 : Integrator  InitialConditionSource=external
  TH1_D : Outport
  TH1 : Outport  Port=2
  wires:
  TH1_DD/1 -> Integrator2/1  "Theta1_DD"
  Constant15/1 -> Integrator3/2
  Constant16/1 -> Integrator2/2
  Integrator3/1 -> TH1/1  "Theta1"
  Integrator2/1 -> TH1_D/1, Integrator3/1  "Theta1_D"

== system bh_4dof_LAGR_manipulator_CONTROL_PID/Variant Subsystem/SIMULINK_MODEL/THETA_2 ==
  TH2_DD : Inport
  Constant15 : Constant  Value=theta2_0
  Constant16 : Constant  Value=theta2_dot_0
  Integrator2 : Integrator  InitialConditionSource=external
  Integrator3 : Integrator  InitialConditionSource=external
  TH2_D : Outport
  TH2 : Outport  Port=2
  wires:
  TH2_DD/1 -> Integrator2/1  "Theta2_DD"
  Integrator2/1 -> TH2_D/1, Integrator3/1  "Theta2_D"
  Constant15/1 -> Integrator3/2
  Constant16/1 -> Integrator2/2
  Integrator3/1 -> TH2/1  "Theta2"

== system bh_4dof_LAGR_manipulator_CONTROL_PID/Variant Subsystem/SIMULINK_MODEL/THETA_3 ==
  TH3_DD : Inport
  Constant15 : Constant  Value=theta3_0
  Constant16 : Constant  Value=theta3_dot_0
  Integrator2 : Integrator  InitialConditionSource=external
  Integrator3 : Integrator  InitialConditionSource=external
  TH3_D : Outport
  TH3 : Outport  Port=2
  wires:
  TH3_DD/1 -> Integrator2/1  "Theta3_DD"
  Integrator2/1 -> TH3_D/1, Integrator3/1  "Theta3_D"
  Constant15/1 -> Integrator3/2
  Constant16/1 -> Integrator2/2
  Integrator3/1 -> TH3/1  "Theta3"

== system bh_4dof_LAGR_manipulator_CONTROL_PID/Variant Subsystem/SIMULINK_MODEL/THETA_4 ==
  TH4_DD : Inport
  Constant15 : Constant  Value=theta4_0
  Constant16 : Constant  Value=theta4_dot_0
  Integrator2 : Integrator  InitialConditionSource=external
  Integrator3 : Integrator  InitialConditionSource=external
  TH4_D : Outport
  TH4 : Outport  Port=2
  wires:
  TH4_DD/1 -> Integrator2/1  "Theta4_DD"
  Integrator2/1 -> TH4_D/1, Integrator3/1  "Theta4_D"
  Constant15/1 -> Integrator3/2
  Constant16/1 -> Integrator2/2
  Integrator3/1 -> TH4/1  "Theta4"

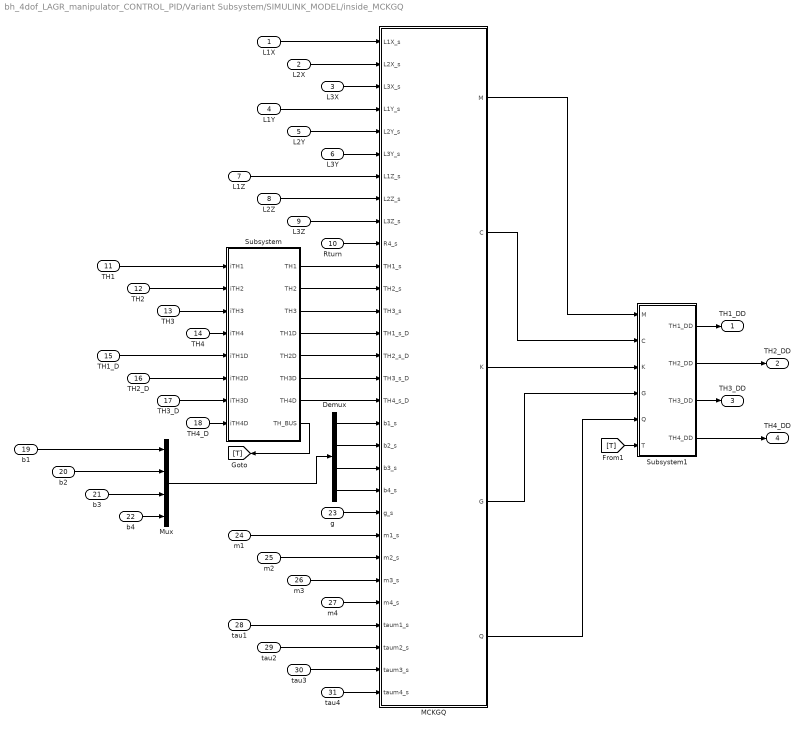
== system bh_4dof_LAGR_manipulator_CONTROL_PID/Variant Subsystem/SIMULINK_MODEL/inside_MCKGQ ==
  L1X : Inport
  L2X : Inport  Port=2
  L3X : Inport  Port=3
  L1Y : Inport  Port=4
  L2Y : Inport  Port=5
  L3Y : Inport  Port=6
  L1Z : Inport  Port=7
  L2Z : Inport  Port=8
  L3Z : Inport  Port=9
  Rturn : Inport  Port=10
  TH1 : Inport  Port=11
  TH2 : Inport  Port=12
  TH3 : Inport  Port=13
  TH4 : Inport  Port=14
  TH1_D : Inport  Port=15
  TH2_D : Inport  Port=16
  TH3_D : Inport  Port=17
  TH4_D : Inport  Port=18
  b1 : Inport  Port=19
  b2 : Inport  Port=20
  b3 : Inport  Port=21
  b4 : Inport  Port=22
  g : Inport  Port=23
  m1 : Inport  Port=24
  m2 : Inport  Port=25
  m3 : Inport  Port=26
  m4 : Inport  Port=27
  tau1 : Inport  Port=28
  tau2 : Inport  Port=29
  tau3 : Inport  Port=30
  tau4 : Inport  Port=31
  Demux : Demux
  MCKGQ : MATLAB Function  TreatAsAtomicUnit=on
  Mux : Mux
  Subsystem : Subsystem
  Subsystem1 : Subsystem
  TH1_DD : Outport
  TH2_DD : Outport  Port=2
  TH3_DD : Outport  Port=3
  TH4_DD : Outport  Port=4
  wires:
  m2/1 -> MCKGQ/24(m2_s)
  m3/1 -> MCKGQ/25(m3_s)
  m4/1 -> MCKGQ/26(m4_s)
  tau1/1 -> MCKGQ/27(taum1_s)
  g/1 -> MCKGQ/22(g_s)
  m1/1 -> MCKGQ/23(m1_s)
  TH1_D/1 -> Subsystem/5(iTH1D)
  b1/1 -> Mux/1
  b2/1 -> Mux/2
  TH3/1 -> Subsystem/3(iTH3)
  b3/1 -> Mux/3
  TH4_D/1 -> Subsystem/8(iTH4D)
  TH2_D/1 -> Subsystem/6(iTH2D)
  TH3_D/1 -> Subsystem/7(iTH3D)
  b4/1 -> Mux/4
  tau2/1 -> MCKGQ/28(taum2_s)
  tau3/1 -> MCKGQ/29(taum3_s)
  tau4/1 -> MCKGQ/30(taum4_s)
  L2X/1 -> MCKGQ/2(L2X_s)
  L3X/1 -> MCKGQ/3(L3X_s)
  L2Y/1 -> MCKGQ/5(L2Y_s)
  L3Y/1 -> MCKGQ/6(L3Y_s)
  L1Y/1 -> MCKGQ/4(L1Y_s)
  L2Z/1 -> MCKGQ/8(L2Z_s)
  L3Z/1 -> MCKGQ/9(L3Z_s)
  L1Z/1 -> MCKGQ/7(L1Z_s)
  TH1/1 -> Subsystem/1(iTH1)
  Rturn/1 -> MCKGQ/10(R4_s)
  TH2/1 -> Subsystem/2(iTH2)
  L1X/1 -> MCKGQ/1(L1X_s)
  Subsystem/8(TH_BUS) -> [T]
  Subsystem/7(TH4D) -> MCKGQ/17(TH4_s_D)
  Subsystem/6(TH3D) -> MCKGQ/16(TH3_s_D)
  Subsystem/5(TH2D) -> MCKGQ/15(TH2_s_D)
  Subsystem/4(TH1D) -> MCKGQ/14(TH1_s_D)
  Subsystem/3(TH3) -> MCKGQ/13(TH3_s)
  Subsystem/2(TH2) -> MCKGQ/12(TH2_s)
  Subsystem/1(TH1) -> MCKGQ/11(TH1_s)
  TH4/1 -> Subsystem/4(iTH4)
  Demux/1 -> MCKGQ/18(b1_s)
  Demux/2 -> MCKGQ/19(b2_s)
  Demux/3 -> MCKGQ/20(b3_s)
  Demux/4 -> MCKGQ/21(b4_s)
  Mux/1 -> Demux/1
  Subsystem1/1(TH1_DD) -> TH1_DD/1
  Subsystem1/2(TH2_DD) -> TH2_DD/1
  MCKGQ/1(M) -> Subsystem1/1(M)
  MCKGQ/2(C) -> Subsystem1/2(C)
  MCKGQ/3(K) -> Subsystem1/3(K)
  MCKGQ/4(G) -> Subsystem1/4(G)
  MCKGQ/5(Q) -> Subsystem1/5(Q)
  [T] -> Subsystem1/6(T)
  Subsystem1/3(TH3_DD) -> TH3_DD/1
  Subsystem1/4(TH4_DD) -> TH4_DD/1

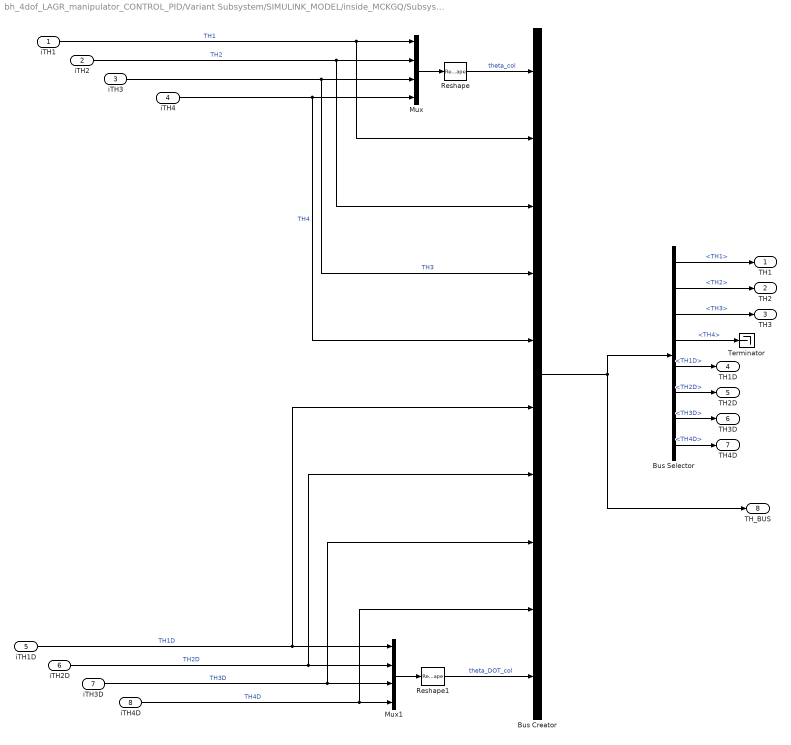
== system bh_4dof_LAGR_manipulator_CONTROL_PID/Variant Subsystem/SIMULINK_MODEL/inside_MCKGQ/Subsystem ==
  iTH1 : Inport
  iTH2 : Inport  Port=2
  iTH3 : Inport  Port=3
  iTH4 : Inport  Port=4
  iTH1D : Inport  Port=5
  iTH2D : Inport  Port=6
  iTH3D : Inport  Port=7
  iTH4D : Inport  Port=8
  Bus Creator : BusCreator  Inputs=10
  Bus Selector : BusSelector  OutputSignals=TH1,TH2,TH3,TH4,TH1D,TH2D,TH3D,TH4D
  Mux : Mux
  Mux1 : Mux
  Reshape : Reshape  OutputDimensionality=Column vector (2-D)
  Reshape1 : Reshape  OutputDimensionality=Column vector (2-D)
  Terminator : Terminator
  TH1 : Outport
  TH2 : Outport  Port=2
  TH3 : Outport  Port=3
  TH1D : Outport  Port=4
  TH2D : Outport  Port=5
  TH3D : Outport  Port=6
  TH4D : Outport  Port=7
  TH_BUS : Outport  Port=8
  wires:
  iTH2/1 -> Bus Creator/3, Mux/2  "TH2"
  iTH1/1 -> Bus Creator/2, Mux/1  "TH1"
  iTH2D/1 -> Bus Creator/7, Mux1/2  "TH2D"
  iTH1D/1 -> Bus Creator/6, Mux1/1  "TH1D"
  Mux/1 -> Reshape/1
  Mux1/1 -> Reshape1/1
  Reshape/1 -> Bus Creator/1  "theta_col"
  Reshape1/1 -> Bus Creator/10  "theta_DOT_col"
  Bus Creator/1 -> TH_BUS/1, Bus Selector/1
  iTH3D/1 -> Bus Creator/8, Mux1/3  "TH3D"
  iTH3/1 -> Bus Creator/4, Mux/3  "TH3"
  Bus Selector/1 -> TH1/1  "<TH1>"
  Bus Selector/2 -> TH2/1  "<TH2>"
  Bus Selector/3 -> TH3/1  "<TH3>"
  Bus Selector/5 -> TH1D/1  "<TH1D>"
  Bus Selector/6 -> TH2D/1  "<TH2D>"
  Bus Selector/7 -> TH3D/1  "<TH3D>"
  iTH4/1 -> Bus Creator/5, Mux/4  "TH4"
  iTH4D/1 -> Bus Creator/9, Mux1/4  "TH4D"
  Bus Selector/4 -> Terminator/1  "<TH4>"
  Bus Selector/8 -> TH4D/1  "<TH4D>"

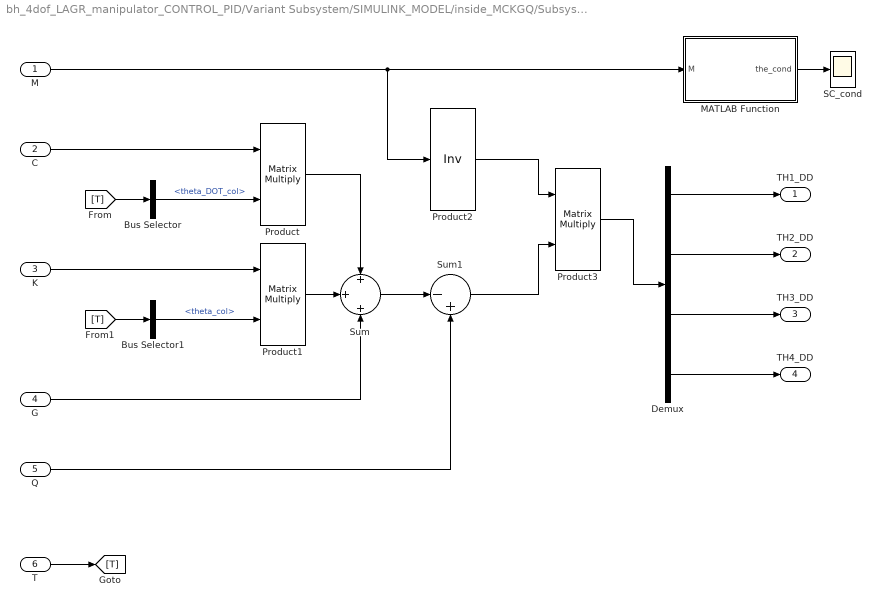
== system bh_4dof_LAGR_manipulator_CONTROL_PID/Variant Subsystem/SIMULINK_MODEL/inside_MCKGQ/Subsystem1 ==
  M : Inport
  C : Inport  Port=2
  K : Inport  Port=3
  G : Inport  Port=4
  Q : Inport  Port=5
  T : Inport  Port=6
  Bus Selector : BusSelector  OutputSignals=theta_DOT_col
  Bus Selector1 : BusSelector  OutputSignals=theta_col
  Demux : Demux
  MATLAB Function : MATLAB Function  TreatAsAtomicUnit=on
  Product : Product  Multiplication=Matrix(*)
  Product1 : Product  Multiplication=Matrix(*)
  Product2 : Product  Inputs=/  Multiplication=Matrix(*)
  Product3 : Product  Multiplication=Matrix(*)
  SC_cond : Scope
  Sum : Sum  Inputs=+|+|+
  Sum1 : Sum  Inputs=|-+
  TH1_DD : Outport
  TH2_DD : Outport  Port=2
  TH3_DD : Outport  Port=3
  TH4_DD : Outport  Port=4
  wires:
  T/1 -> [T]
  C/1 -> Product/1
  [T] -> Bus Selector/1
  Bus Selector/1 -> Product/2  "<theta_DOT_col>"
  K/1 -> Product1/1
  [T] -> Bus Selector1/1
  Bus Selector1/1 -> Product1/2  "<theta_col>"
  Q/1 -> Sum1/2
  Product1/1 -> Sum/2
  G/1 -> Sum/3
  Product/1 -> Sum/1
  Sum/1 -> Sum1/1
  M/1 -> Product2/1, MATLAB Function/1(M)
  Product2/1 -> Product3/1
  Sum1/1 -> Product3/2
  Product3/1 -> Demux/1
  Demux/1 -> TH1_DD/1
  Demux/2 -> TH2_DD/1
  MATLAB Function/1(the_cond) -> SC_cond/1
  Demux/3 -> TH3_DD/1
  Demux/4 -> TH4_DD/1

== matlab function bh_4dof_LAGR_manipulator_CONTROL_PID/TRAJECTORY/THE_J ==
  data: L1Y_s input; the_J output; L2Y_s input; L3Y_s input; theta1 input; theta2 input; theta3 input; theta4 input
function the_J = THE_J(L1Y_s,L2Y_s,L3Y_s,theta1,theta2,theta3,theta4)
%#codegen

%    This function was generated by the Symbolic Math Toolbox version 7.0.
%    13-Sep-2016 14:49:06

the_J = reshape([sin(theta4).*(L2Y_s.*sin(theta1+theta2)+L1Y_s.*sin(theta1)+L3Y_s.*sin(theta1+theta2+theta3)),-cos(theta4).*(L2Y_s.*sin(theta1+theta2)+L1Y_s.*sin(theta1)+L3Y_s.*sin(theta1+theta2+theta3)),L2Y_s.*cos(theta1+theta2)+L1Y_s.*cos(theta1)+L3Y_s.*cos(theta1+theta2+theta3),sin(theta4).*(L2Y_s.*sin(theta1+theta2)+L3Y_s.*sin(theta1+theta2+theta3)),-cos(theta4).*(L2Y_s.*sin(theta1+theta2)+L3Y_s.*sin(theta1+theta2+theta3)),L2Y_s.*cos(theta1+theta2)+L3Y_s.*cos(theta1+theta2+theta3),L3Y_s.*sin(theta1+theta2+theta3).*sin(theta4),-L3Y_s.*sin(theta1+theta2+theta3).*cos(theta4),L3Y_s.*cos(theta1+theta2+theta3),-cos(theta4).*(L2Y_s.*cos(theta1+theta2)+L1Y_s.*cos(theta1)+L3Y_s.*cos(theta1+theta2+theta3)),-sin(theta4).*(L2Y_s.*cos(theta1+theta2)+L1Y_s.*cos(theta1)+L3Y_s.*cos(theta1+theta2+theta3)),0.0],[3,4]);
